simulink library "dac"  (Simulink 6.2)
settings Model: LastModifiedBy=rolf

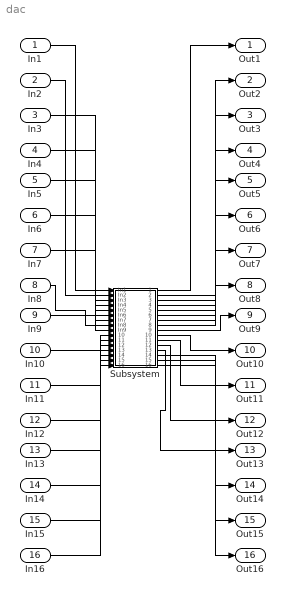
== system dac ==
  In1 : Inport  Port=1  LatchInput=off
  In2 : Inport  Port=2  LatchInput=off
  In3 : Inport  Port=3  LatchInput=off
  In4 : Inport  Port=4  LatchInput=off
  In5 : Inport  Port=5  LatchInput=off
  In6 : Inport  Port=6  LatchInput=off
  In7 : Inport  Port=7  LatchInput=off
  In8 : Inport  Port=8  LatchInput=off
  In9 : Inport  Port=9  LatchInput=off
  In10 : Inport  Port=10  LatchInput=off
  In11 : Inport  Port=11  LatchInput=off
  In12 : Inport  Port=12  LatchInput=off
  In13 : Inport  Port=13  LatchInput=off
  In14 : Inport  Port=14  LatchInput=off
  In15 : Inport  Port=15  LatchInput=off
  In16 : Inport  Port=16  LatchInput=off
  Subsystem : Subsystem
  Out1 : Outport
  Out2 : Outport  Port=2
  Out3 : Outport  Port=3
  Out4 : Outport  Port=4
  Out5 : Outport  Port=5
  Out6 : Outport  Port=6
  Out7 : Outport  Port=7
  Out8 : Outport  Port=8
  Out9 : Outport  Port=9
  Out10 : Outport  Port=10
  Out11 : Outport  Port=11
  Out12 : Outport  Port=12
  Out13 : Outport  Port=13
  Out14 : Outport  Port=14
  Out15 : Outport  Port=15
  Out16 : Outport  Port=16
  wires:
  Subsystem/1(Out1) -> Out1/1
  In1/1 -> Subsystem/1(In1)
  Subsystem/2(Out2) -> Out2/1
  In2/1 -> Subsystem/2(In2)
  Subsystem/3(Out3) -> Out3/1
  In3/1 -> Subsystem/3(In3)
  Subsystem/4(Out4) -> Out4/1
  In4/1 -> Subsystem/4(In4)
  Subsystem/5(Out5) -> Out5/1
  In5/1 -> Subsystem/5(In5)
  Subsystem/6(Out6) -> Out6/1
  In6/1 -> Subsystem/6(In6)
  Subsystem/7(Out7) -> Out7/1
  In7/1 -> Subsystem/7(In7)
  Subsystem/8(Out8) -> Out8/1
  In8/1 -> Subsystem/8(In8)
  Subsystem/9(Out9) -> Out9/1
  In9/1 -> Subsystem/9(In9)
  Subsystem/10(Out10) -> Out10/1
  In10/1 -> Subsystem/10(In10)
  Subsystem/11(Out11) -> Out11/1
  In11/1 -> Subsystem/11(In11)
  Subsystem/12(Out12) -> Out12/1
  In12/1 -> Subsystem/12(In12)
  Subsystem/13(Out13) -> Out13/1
  In13/1 -> Subsystem/13(In13)
  Subsystem/14(Out14) -> Out14/1
  In14/1 -> Subsystem/14(In14)
  Subsystem/15(Out15) -> Out15/1
  In15/1 -> Subsystem/15(In15)
  Subsystem/16(Out16) -> Out16/1
  In16/1 -> Subsystem/16(In16)

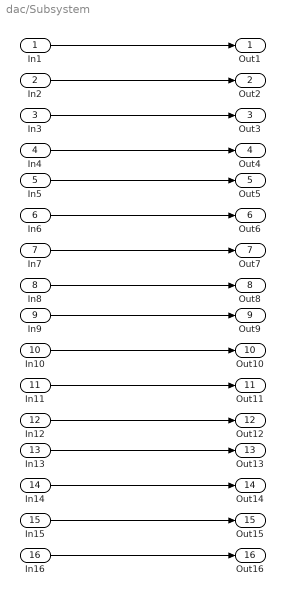
== system dac/Subsystem ==
  In1 : Inport  Port=1  LatchInput=off
  In2 : Inport  Port=2  LatchInput=off
  In3 : Inport  Port=3  LatchInput=off
  In4 : Inport  Port=4  LatchInput=off
  In5 : Inport  Port=5  LatchInput=off
  In6 : Inport  Port=6  LatchInput=off
  In7 : Inport  Port=7  LatchInput=off
  In8 : Inport  Port=8  LatchInput=off
  In9 : Inport  Port=9  LatchInput=off
  In10 : Inport  Port=10  LatchInput=off
  In11 : Inport  Port=11  LatchInput=off
  In12 : Inport  Port=12  LatchInput=off
  In13 : Inport  Port=13  LatchInput=off
  In14 : Inport  Port=14  LatchInput=off
  In15 : Inport  Port=15  LatchInput=off
  In16 : Inport  Port=16  LatchInput=off
  Out1 : Outport
  Out2 : Outport  Port=2
  Out3 : Outport  Port=3
  Out4 : Outport  Port=4
  Out5 : Outport  Port=5
  Out6 : Outport  Port=6
  Out7 : Outport  Port=7
  Out8 : Outport  Port=8
  Out9 : Outport  Port=9
  Out10 : Outport  Port=10
  Out11 : Outport  Port=11
  Out12 : Outport  Port=12
  Out13 : Outport  Port=13
  Out14 : Outport  Port=14
  Out15 : Outport  Port=15
  Out16 : Outport  Port=16
  wires:
  In1/1 -> Out1/1
  In2/1 -> Out2/1
  In3/1 -> Out3/1
  In4/1 -> Out4/1
  In5/1 -> Out5/1
  In6/1 -> Out6/1
  In7/1 -> Out7/1
  In8/1 -> Out8/1
  In9/1 -> Out9/1
  In10/1 -> Out10/1
  In11/1 -> Out11/1
  In12/1 -> Out12/1
  In13/1 -> Out13/1
  In14/1 -> Out14/1
  In15/1 -> Out15/1
  In16/1 -> Out16/1
